simulink model "wirkungsplan_mdl"  (R2013b)
settings: Solver=ode45  StartTime=0.0  StopTime=0.5  MaxStep=1e-5  RelTol=1e-3
values from neighbouring files (symbols this model uses):
  a = 0.001    [wirkungsplan.m]
  J = 44e-7 + 1e-5    (= 1.44e-05)    [wirkungsplan.m]
  Kw = 1/250    (= 0.004)    [wirkungsplan.m]
  L = 1.04e-3    (= 0.00104)    [wirkungsplan.m]
  Ml = 0    [wirkungsplan.m]
  R = 7.19    [wirkungsplan.m]
settings Model: Creator=daniw  LastModifiedBy=daniw

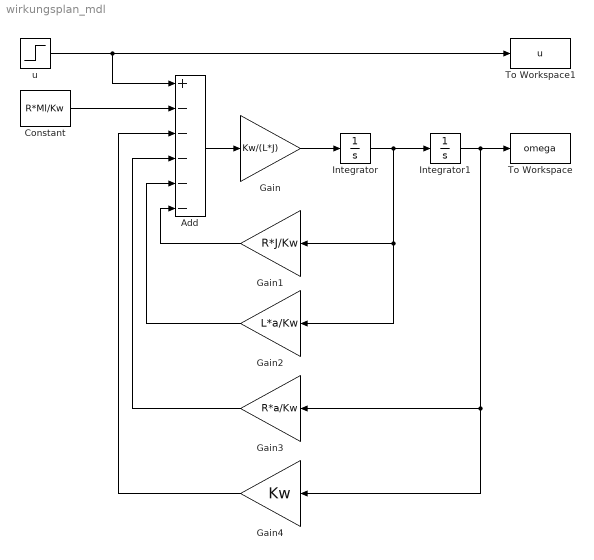
== system wirkungsplan_mdl ==
  Add : Sum  Inputs=+-----
  Constant : Constant  Value=R*Ml/Kw
  Gain : Gain  Gain=Kw/(L*J)
  Gain1 : Gain  Gain=R*J/Kw
  Gain2 : Gain  Gain=L*a/Kw
  Gain3 : Gain  Gain=R*a/Kw
  Gain4 : Gain  Gain=Kw
  Integrator : Integrator
  Integrator1 : Integrator
  To Workspace : ToWorkspace  VariableName=omega  SampleTime=-1  SaveFormat=Structure With Time
  To Workspace1 : ToWorkspace  VariableName=u  SampleTime=-1  SaveFormat=Structure With Time
  u : Step  Time=0.01  SampleTime=0
  wires:
  u/1 -> To Workspace1/1, Add/1
  Add/1 -> Gain/1
  Integrator/1 -> Gain2/1, Gain1/1, Integrator1/1
  Gain/1 -> Integrator/1
  Constant/1 -> Add/2
  Gain1/1 -> Add/6
  Gain2/1 -> Add/5
  Gain3/1 -> Add/4
  Gain4/1 -> Add/3
  Integrator1/1 -> Gain4/1, Gain3/1, To Workspace/1
